simulink model "assignment1"  (R2019a)
settings: Solver=FixedStepDiscrete  StartTime=0.0  StopTime=10.0  RelTol=1e-3
libraries: simulink x4
settings Model: Creator=INDIA  LastModifiedBy=INDIA

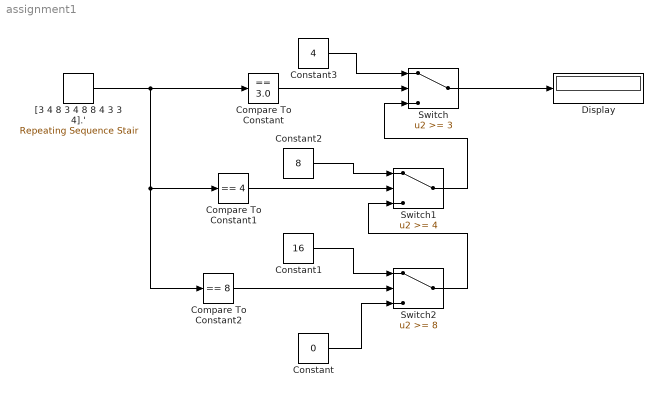
== system assignment1 ==
  Compare To Constant : simulink/Logic and Bit Operations/Compare To Constant  relop===  const=3.0  OutDataTypeStr=boolean
  Compare To Constant1 : simulink/Logic and Bit Operations/Compare To Constant  relop===  const=4  OutDataTypeStr=boolean
  Compare To Constant2 : simulink/Logic and Bit Operations/Compare To Constant  relop===  const=8  OutDataTypeStr=boolean
  Constant : Constant  Value=0
  Constant1 : Constant  Value=16
  Constant2 : Constant  Value=8
  Constant3 : Constant  Value=4
  Display : Display
  Switch : Switch  Threshold=3
  Switch1 : Switch  Threshold=4
  Switch2 : Switch  Threshold=8
  "[3 4 8 3 4 8 8 4 3 3 4].'" : simulink/Sources/Repeating Sequence Stair  OutValues=[3 4 8 3 4 8 8 4 3 3 4].'  tsamp=-1  OutMin=[]  OutMax=[]  OutDataTypeStr=double  OutputDataTypeScalingMode=double  OutDataType=fixdt(0,8)  ConRadixGroup=Best Precision: Vector-wise  OutScaling=2^-12
  wires:
  Switch1/1 -> Switch/3
  Switch2/1 -> Switch1/3
  "[3 4 8 3 4 8 8 4 3 3 4].'"/1 -> Compare To Constant2/1, Compare To Constant1/1, Compare To Constant/1
  Constant/1 -> Switch2/3
  Switch/1 -> Display/1
  Constant1/1 -> Switch2/1
  Constant3/1 -> Switch/1
  Constant2/1 -> Switch1/1
  Compare To Constant/1 -> Switch/2
  Compare To Constant1/1 -> Switch1/2
  Compare To Constant2/1 -> Switch2/2
